simulink model "step_response"  (R2021a)
settings: Solver=FixedStepAuto  StartTime=0.0  StopTime=Inf  FixedStep=0.01  RelTol=1e-3  EnableMultiTasking=on
libraries: arduinolib x4, simulink x2
settings Model: SILPILModeSetting=veronly  ExtModeTrigDuration=2  Creator=Simón  LastModifiedBy=Simón
settings OptimizationCC: EnhancedBackFolding=on  PassReuseOutputArgsAs=Individual arguments  ZeroExternalMemoryAtStartup=off  ZeroInternalMemoryAtStartup=off  MaxStackSize=64  OptimizeBlockOrder=speed  DifferentSizesBufferReuse=on  OptimizationCustomize=off  EfficientTunableParamExpr=on
settings DebuggingCC: ParameterTunabilityLossMsg=error
settings HardwareCC: ProdBitPerInt=16  ProdBitPerPointer=16  ProdBitPerSizeT=16  ProdBitPerPtrDiffT=16  ProdLargestAtomicFloat=None  ProdWordSize=8  ProdHWDeviceType=Atmel->AVR  UseEmbeddedCoderFeatures=off  UseSimulinkCoderFeatures=off
settings SFSimCC: MATLABDynamicMemAlloc=off
settings RTWCC: SystemTargetFile=ert.tlc  HardwareBoard=Arduino Uno  TemplateMakefile=ert_default_tmf  Toolchain=Arduino AVR  BuildConfiguration=Faster Runs
settings CodeAppCC: ForceParamTrailComments=on  IgnoreCustomStorageClasses=off  OperatorAnnotations=on  SimulinkDataObjDesc=on  SFDataObjDesc=on  InsertBlockDesc=on
settings ERTTargetCC: SupportContinuousTime=on  SupportNonInlinedSFcns=on  SupportVariableSizeSignals=on  ExtModeStaticAllocSize=250

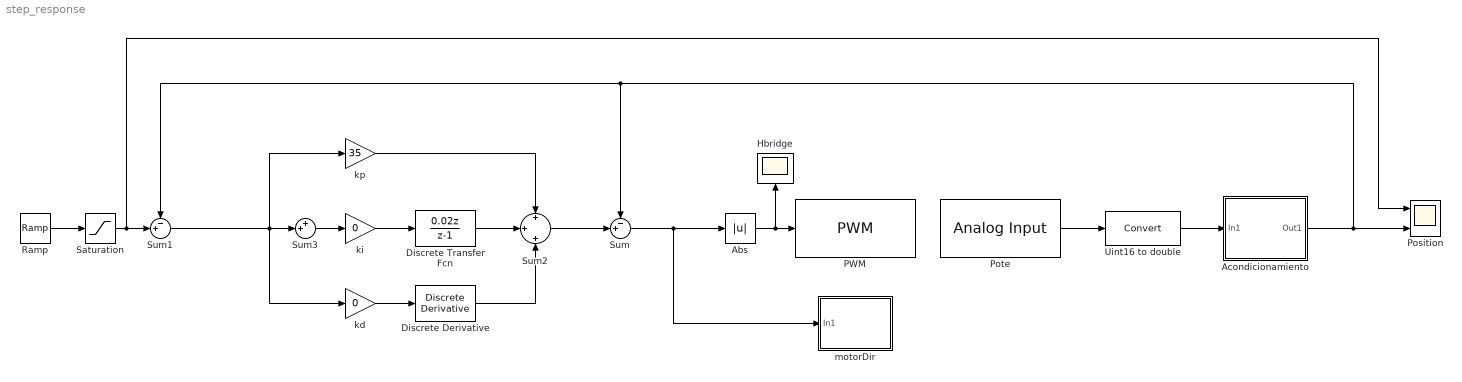
== system step_response ==
  Abs : Abs
  Acondicionamiento : Subsystem
  Discrete Transfer Fcn : DiscreteTransferFcn  Numerator=[0.02 0]  Denominator=[1 -1]
  Discrete Derivative : simulink/Discrete/Discrete Derivative  gainval=1.0  ICPrevScaledInput=0.0  OutMin=[]  OutMax=[]  OutDataType=fixdt(1, 16)  OutScaling=2^-10  DoSatur=off
  Hbridge : Scope
  PWM : arduinolib/PWM  pinNumber=10  frequencyType=Default  desiredFrequency=490.2  achievableFrequency=490.2
  Position : Scope  NumInputPorts=2
  Pote : arduinolib/Analog Input  pinNumber=0  ReadResultsOnly=off  ConversionTriggerSource=Software  ExternalTriggerType=uint32( 0 )  OutputDataType=uint16  EnableConversionCompleteNotify=off  EnableOuputStatus=off  SampleTime=-1  blockPlatform=arduino
  Ramp : simulink/Sources/Ramp  slope=50  start=0  InitialOutput=0
  Saturation : Saturate  UpperLimit=80  LowerLimit=0
  Sum : Sum  Inputs=-+|
  Sum1 : Sum  Inputs=-+|
  Sum2 : Sum  Inputs=+|+|+
  Sum3 : Sum  Inputs=++|
  Uint16 to double : DataTypeConversion
  kd : Gain  Gain=0
  ki : Gain  Gain=0
  kp : Gain  Gain=35
  motorDir : Subsystem
  wires:
  Pote/1 -> Uint16 to double/1
  Uint16 to double/1 -> Acondicionamiento/1(In1)
  Sum/1 -> Abs/1, motorDir/1(In1)
  Acondicionamiento/1(Out1) -> Position/2, Sum1/1, Sum/1
  Abs/1 -> Hbridge/1, PWM/1
  kd/1 -> Discrete Derivative/1
  Discrete Derivative/1 -> Sum2/3
  Sum1/1 -> Sum3/2, kp/1, kd/1
  kp/1 -> Sum2/1
  Sum2/1 -> Sum/2
  Discrete Transfer Fcn/1 -> Sum2/2
  ki/1 -> Discrete Transfer Fcn/1
  Ramp/1 -> Saturation/1
  Sum3/1 -> ki/1
  Saturation/1 -> Position/1, Sum1/2

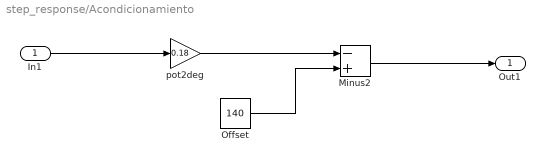
== system step_response/Acondicionamiento ==
  In1 : Inport
  Minus2 : Sum  Inputs=-+
  Offset : Constant  Value=140
  pot2deg : Gain  Gain=0.18
  Out1 : Outport
  wires:
  Offset/1 -> Minus2/2
  pot2deg/1 -> Minus2/1
  Minus2/1 -> Out1/1
  In1/1 -> pot2deg/1

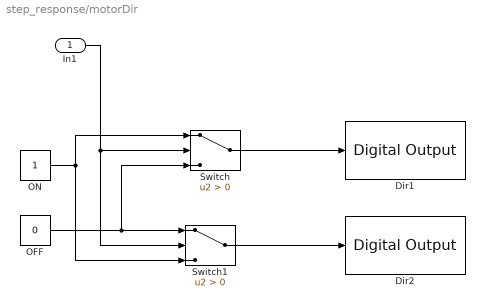
== system step_response/motorDir ==
  In1 : Inport
  Dir1 : arduinolib/Digital Output  pinNumber=8  Direction=output  blockPlatform=arduino
  Dir2 : arduinolib/Digital Output  pinNumber=9  Direction=output  blockPlatform=arduino
  OFF : Constant  Value=0
  ON : Constant
  Switch : Switch  Criteria=u2 > Threshold
  Switch1 : Switch  Criteria=u2 > Threshold
  wires:
  In1/1 -> Switch1/2, Switch/2
  OFF/1 -> Switch/3, Switch1/1
  ON/1 -> Switch1/3, Switch/1
  Switch1/1 -> Dir2/1
  Switch/1 -> Dir1/1
